simulink model "SigProcess"  (R2022b)
settings: Solver=FixedStepDiscrete  StartTime=0.0  StopTime=10.0  FixedStep=0.001  RelTol=1e-3
undefined symbols (not defined in the file): cClCddAdc_D_u16ADNum, cClCddAdc_D_u8FilterType, cClCddAdc_D_u8RawValueNum, cTmAfCtrl_Te_s32ShttrPosnColdOnHp
libraries: simulink x132
(part 7 of 7)

== system SigProcess/SigProcessSub/Stp5_ChangeAttrAndName/3_createPortGotoUpdate2/31_AdFilter/319_AVG5 ==
  sigin : Inport
  3191_MATLAB Function : MATLAB Function  TreatAsAtomicUnit=on
  Compare To Constant : simulink/Logic and Bit Operations/Compare To Constant  relop===  const=0  OutDataTypeStr=boolean
  Constant : Constant  Value=cClCddAdc_D_u8FilterType  OutDataTypeStr=uint8
  Constant1 : Constant  Value=cClCddAdc_D_u8RawValueNum  OutDataTypeStr=uint8
  Counter Limited : simulink/Sources/Counter Limited  uplimit=cClCddAdc_D_u8RawValueNum-1  tsamp=-1
  Data Store Memory : DataStoreMemory  DataStoreName=RecFlapFbRaw  ReadBeforeWriteMsg=warning  WriteAfterWriteMsg=warning  WriteAfterReadMsg=warning  ShowAdditionalParam=off  OutDataTypeStr=single  Dimensions=[1 20]
      settings: CopyFcn=set_param(gcbh,'ShowName','off');
  Data Store Read : DataStoreRead  DataStoreName=RecFlapFbRaw  IndexOptions=Index vector (dialog)  Indices=1  OutputSizes=1
  Data Store Write : DataStoreWrite  DataStoreName=RecFlapFbRaw  DataStoreElements=RecFlapFbRaw  EnableIndexing=on  IndexMode=Zero-based  IndexOptions=Index vector (port)  Indices=1  OutputSizes=1
  Data Type Conversion : DataTypeConversion  OutDataTypeStr=single  SaturateOnIntegerOverflow=off  RndMeth=Floor
  Gain1 : Gain  Gain=1/cClCddAdc_D_u8RawValueNum
  Multiport Switch : MultiPortSwitch  DataPortOrder=Zero-based contiguous  Inputs=5  DataPortForDefault=Additional data port  zeroidx=on  OutDataTypeStr=single  SaturateOnIntegerOverflow=off  InputSameDT=off
  Scope : Scope
  Sum of Elements1 : Sum  Inputs=+
  Switch : Switch  Criteria=u2 ~= 0  SaturateOnIntegerOverflow=off  InputSameDT=off
  Unit Delay : UnitDelay  SampleTime=-1  HasFrameUpgradeWarning=on
  sigAvg : Outport  OutDataTypeStr=single
  wires:
  Constant1/1 -> 3191_MATLAB Function/2(num)
  [sigAvg] -> sigAvg/1
  Multiport Switch/1 -> [sigAvg]
  [siginSingle] -> Multiport Switch/2
  [sigAvgQuick] -> Multiport Switch/6
  [sigAvgSimple] -> Multiport Switch/5
  [sigAvgSortWithoutEdge] -> Multiport Switch/4
  [sigAvgSortedMid] -> Multiport Switch/3
  Constant/1 -> Multiport Switch/1
  [sigin] -> Multiport Switch/7
  [sigin] -> Data Type Conversion/1
  sigin/1 -> [sigin]
  3191_MATLAB Function/1(mid) -> [sigAvgSortedMid]
  Unit Delay/1 -> Switch/3
  3191_MATLAB Function/2(withoutEdge) -> [sigAvgSortWithoutEdge]
  Data Type Conversion/1 -> Scope/1, Data Store Write/1, [siginSingle]
  Counter Limited/1 -> Data Store Write/2, Compare To Constant/1
  Gain1/1 -> [sigAvgQuick], Switch/1
  Switch/1 -> Unit Delay/1, [sigAvgSimple]
  Compare To Constant/1 -> Switch/2
  Sum of Elements1/1 -> Gain1/1
  Data Store Read/1 -> Sum of Elements1/1, 3191_MATLAB Function/1(u)

== system SigProcess/SigProcessSub/Stp5_ChangeAttrAndName/1_createPortGotoUpdate/11_AdFilter/113_AVG/1131_Ad2Volt ==
  ad : Inport
  Gain : Gain  Gain=5/cClCddAdc_D_u16ADNum
  volt : Outport
  wires:
  ad/1 -> Gain/1
  Gain/1 -> volt/1

== system SigProcess/SigProcessSub/Stp5_ChangeAttrAndName/2_createPortGotoUpdate1/21_AdFilter/213_AVG/2131_Ad2Volt ==
  ad : Inport
  Gain : Gain  Gain=5/cClCddAdc_D_u16ADNum
  volt : Outport
  wires:
  Gain/1 -> volt/1
  ad/1 -> Gain/1

== system SigProcess/SigProcessSub/Stp5_ChangeAttrAndName/3_createPortGotoUpdate2/31_AdFilter/313_AVG/3131_Ad2Volt ==
  ad : Inport
  Gain : Gain  Gain=5/cClCddAdc_D_u16ADNum
  volt : Outport
  wires:
  ad/1 -> Gain/1
  Gain/1 -> volt/1

== matlab function SigProcess/SigProcessSub/Stp3_createGotoUpdate/CLHB02001_AdFilter/AVG1/MATLAB Function ==
  data: u input; mid output; withoutEdge output; num input

function [mid, withoutEdge] = fcn(u,num)
% 输入u: 待排序数组
% 输入num: 滤波个数，max is 20
n = num;
for i = 1:n-1
    for j = 1:n-i
        if u(j) > u(j+1)
            temp = u(j);
            u(j) = u(j+1);
            u(j+1) = temp;
        end
    end
end
sortedData = u;

mid = sortedData(ceil(num/2)); % 取中间值
withoutEdge = mean(sortedData(2:num-1));

== matlab function SigProcess/SigProcessSub/Stp3_createGotoUpdate/CLHB02001_AdFilter/AVG10/MATLAB Function ==
  data: u input; mid output; withoutEdge output; num input

function [mid, withoutEdge] = fcn(u,num)
% 输入u: 待排序数组
% 输入num: 滤波个数，max is 20
n = num;
for i = 1:n-1
    for j = 1:n-i
        if u(j) > u(j+1)
            temp = u(j);
            u(j) = u(j+1);
            u(j+1) = temp;
        end
    end
end
sortedData = u;

mid = sortedData(ceil(num/2)); % 取中间值
withoutEdge = mean(sortedData(2:num-1));

== matlab function SigProcess/SigProcessSub/Stp4_createSubModInfo/CLHB02001_AdFilter/AVG/MATLAB Function ==
  data: u input; mid output; withoutEdge output; num input

function [mid, withoutEdge] = fcn(u,num)
% 输入u: 待排序数组
% 输入num: 滤波个数，max is 20
n = num;
for i = 1:n-1
    for j = 1:n-i
        if u(j) > u(j+1)
            temp = u(j);
            u(j) = u(j+1);
            u(j+1) = temp;
        end
    end
end
sortedData = u;

mid = sortedData(ceil(num/2)); % 取中间值
withoutEdge = mean(sortedData(2:num-1));

== matlab function SigProcess/SigProcessSub/Stp4_createSubModInfo/CLHB02001_AdFilter/AVG1/MATLAB Function ==
  data: u input; mid output; withoutEdge output; num input

function [mid, withoutEdge] = fcn(u,num)
% 输入u: 待排序数组
% 输入num: 滤波个数，max is 20
n = num;
for i = 1:n-1
    for j = 1:n-i
        if u(j) > u(j+1)
            temp = u(j);
            u(j) = u(j+1);
            u(j+1) = temp;
        end
    end
end
sortedData = u;

mid = sortedData(ceil(num/2)); % 取中间值
withoutEdge = mean(sortedData(2:num-1));

== matlab function SigProcess/SigProcessSub/Stp4_createSubModInfo/CLHB02001_AdFilter/AVG10/MATLAB Function ==
  data: u input; mid output; withoutEdge output; num input

function [mid, withoutEdge] = fcn(u,num)
% 输入u: 待排序数组
% 输入num: 滤波个数，max is 20
n = num;
for i = 1:n-1
    for j = 1:n-i
        if u(j) > u(j+1)
            temp = u(j);
            u(j) = u(j+1);
            u(j+1) = temp;
        end
    end
end
sortedData = u;

mid = sortedData(ceil(num/2)); % 取中间值
withoutEdge = mean(sortedData(2:num-1));

== matlab function SigProcess/SigProcessSub/Stp4_createSubModInfo/CLHB02001_AdFilter/AVG2/MATLAB Function ==
  data: u input; mid output; withoutEdge output; num input

function [mid, withoutEdge] = fcn(u,num)
% 输入u: 待排序数组
% 输入num: 滤波个数，max is 20
n = num;
for i = 1:n-1
    for j = 1:n-i
        if u(j) > u(j+1)
            temp = u(j);
            u(j) = u(j+1);
            u(j+1) = temp;
        end
    end
end
sortedData = u;

mid = sortedData(ceil(num/2)); % 取中间值
withoutEdge = mean(sortedData(2:num-1));

== matlab function SigProcess/SigProcessSub/Stp4_createSubModInfo/CLHB02001_AdFilter/AVG3/MATLAB Function ==
  data: u input; mid output; withoutEdge output; num input

function [mid, withoutEdge] = fcn(u,num)
% 输入u: 待排序数组
% 输入num: 滤波个数，max is 20
n = num;
for i = 1:n-1
    for j = 1:n-i
        if u(j) > u(j+1)
            temp = u(j);
            u(j) = u(j+1);
            u(j+1) = temp;
        end
    end
end
sortedData = u;

mid = sortedData(ceil(num/2)); % 取中间值
withoutEdge = mean(sortedData(2:num-1));

== matlab function SigProcess/SigProcessSub/Stp4_createSubModInfo/CLHB02001_AdFilter/AVG4/MATLAB Function ==
  data: u input; mid output; withoutEdge output; num input

function [mid, withoutEdge] = fcn(u,num)
% 输入u: 待排序数组
% 输入num: 滤波个数，max is 20
n = num;
for i = 1:n-1
    for j = 1:n-i
        if u(j) > u(j+1)
            temp = u(j);
            u(j) = u(j+1);
            u(j+1) = temp;
        end
    end
end
sortedData = u;

mid = sortedData(ceil(num/2)); % 取中间值
withoutEdge = mean(sortedData(2:num-1));

== matlab function SigProcess/SigProcessSub/Stp4_createSubModInfo/CLHB02001_AdFilter/AVG5/MATLAB Function ==
  data: u input; mid output; withoutEdge output; num input

function [mid, withoutEdge] = fcn(u,num)
% 输入u: 待排序数组
% 输入num: 滤波个数，max is 20
n = num;
for i = 1:n-1
    for j = 1:n-i
        if u(j) > u(j+1)
            temp = u(j);
            u(j) = u(j+1);
            u(j+1) = temp;
        end
    end
end
sortedData = u;

mid = sortedData(ceil(num/2)); % 取中间值
withoutEdge = mean(sortedData(2:num-1));

== matlab function SigProcess/SigProcessSub/Stp4_createSubModInfo/CLHB02001_AdFilter/AVG6/MATLAB Function ==
  data: u input; mid output; withoutEdge output; num input

function [mid, withoutEdge] = fcn(u,num)
% 输入u: 待排序数组
% 输入num: 滤波个数，max is 20
n = num;
for i = 1:n-1
    for j = 1:n-i
        if u(j) > u(j+1)
            temp = u(j);
            u(j) = u(j+1);
            u(j+1) = temp;
        end
    end
end
sortedData = u;

mid = sortedData(ceil(num/2)); % 取中间值
withoutEdge = mean(sortedData(2:num-1));

== matlab function SigProcess/SigProcessSub/Stp4_createSubModInfo/CLHB02001_AdFilter/AVG7/MATLAB Function ==
  data: u input; mid output; withoutEdge output; num input

function [mid, withoutEdge] = fcn(u,num)
% 输入u: 待排序数组
% 输入num: 滤波个数，max is 20
n = num;
for i = 1:n-1
    for j = 1:n-i
        if u(j) > u(j+1)
            temp = u(j);
            u(j) = u(j+1);
            u(j+1) = temp;
        end
    end
end
sortedData = u;

mid = sortedData(ceil(num/2)); % 取中间值
withoutEdge = mean(sortedData(2:num-1));

== matlab function SigProcess/SigProcessSub/Stp3_createGotoUpdate/CLHB02001_AdFilter/AVG/MATLAB Function ==
  data: u input; mid output; withoutEdge output; num input

function [mid, withoutEdge] = fcn(u,num)
% 输入u: 待排序数组
% 输入num: 滤波个数，max is 20
n = num;
for i = 1:n-1
    for j = 1:n-i
        if u(j) > u(j+1)
            temp = u(j);
            u(j) = u(j+1);
            u(j+1) = temp;
        end
    end
end
sortedData = u;

mid = sortedData(ceil(num/2)); % 取中间值
withoutEdge = mean(sortedData(2:num-1));

== matlab function SigProcess/SigProcessSub/Stp4_createSubModInfo/CLHB02001_AdFilter/AVG8/MATLAB Function ==
  data: u input; mid output; withoutEdge output; num input

function [mid, withoutEdge] = fcn(u,num)
% 输入u: 待排序数组
% 输入num: 滤波个数，max is 20
n = num;
for i = 1:n-1
    for j = 1:n-i
        if u(j) > u(j+1)
            temp = u(j);
            u(j) = u(j+1);
            u(j+1) = temp;
        end
    end
end
sortedData = u;

mid = sortedData(ceil(num/2)); % 取中间值
withoutEdge = mean(sortedData(2:num-1));

== matlab function SigProcess/SigProcessSub/Stp4_createSubModInfo/CLHB02001_AdFilter/AVG9/MATLAB Function ==
  data: u input; mid output; withoutEdge output; num input

function [mid, withoutEdge] = fcn(u,num)
% 输入u: 待排序数组
% 输入num: 滤波个数，max is 20
n = num;
for i = 1:n-1
    for j = 1:n-i
        if u(j) > u(j+1)
            temp = u(j);
            u(j) = u(j+1);
            u(j+1) = temp;
        end
    end
end
sortedData = u;

mid = sortedData(ceil(num/2)); % 取中间值
withoutEdge = mean(sortedData(2:num-1));

== matlab function SigProcess/SigProcessSub/Stp6_createPortGotoUpdate/CLHB02001_AdFilter/AVG/MATLAB Function ==
  data: u input; mid output; withoutEdge output; num input

function [mid, withoutEdge] = fcn(u,num)
% 输入u: 待排序数组
% 输入num: 滤波个数，max is 20
n = num;
for i = 1:n-1
    for j = 1:n-i
        if u(j) > u(j+1)
            temp = u(j);
            u(j) = u(j+1);
            u(j+1) = temp;
        end
    end
end
sortedData = u;

mid = sortedData(ceil(num/2)); % 取中间值
withoutEdge = mean(sortedData(2:num-1));

== matlab function SigProcess/SigProcessSub/Stp6_createPortGotoUpdate/CLHB02001_AdFilter/AVG1/MATLAB Function ==
  data: u input; mid output; withoutEdge output; num input

function [mid, withoutEdge] = fcn(u,num)
% 输入u: 待排序数组
% 输入num: 滤波个数，max is 20
n = num;
for i = 1:n-1
    for j = 1:n-i
        if u(j) > u(j+1)
            temp = u(j);
            u(j) = u(j+1);
            u(j+1) = temp;
        end
    end
end
sortedData = u;

mid = sortedData(ceil(num/2)); % 取中间值
withoutEdge = mean(sortedData(2:num-1));

== matlab function SigProcess/SigProcessSub/Stp6_createPortGotoUpdate/CLHB02001_AdFilter/AVG10/MATLAB Function ==
  data: u input; mid output; withoutEdge output; num input

function [mid, withoutEdge] = fcn(u,num)
% 输入u: 待排序数组
% 输入num: 滤波个数，max is 20
n = num;
for i = 1:n-1
    for j = 1:n-i
        if u(j) > u(j+1)
            temp = u(j);
            u(j) = u(j+1);
            u(j+1) = temp;
        end
    end
end
sortedData = u;

mid = sortedData(ceil(num/2)); % 取中间值
withoutEdge = mean(sortedData(2:num-1));

== matlab function SigProcess/SigProcessSub/Stp6_createPortGotoUpdate/CLHB02001_AdFilter/AVG2/MATLAB Function ==
  data: u input; mid output; withoutEdge output; num input

function [mid, withoutEdge] = fcn(u,num)
% 输入u: 待排序数组
% 输入num: 滤波个数，max is 20
n = num;
for i = 1:n-1
    for j = 1:n-i
        if u(j) > u(j+1)
            temp = u(j);
            u(j) = u(j+1);
            u(j+1) = temp;
        end
    end
end
sortedData = u;

mid = sortedData(ceil(num/2)); % 取中间值
withoutEdge = mean(sortedData(2:num-1));

== matlab function SigProcess/SigProcessSub/Stp6_createPortGotoUpdate/CLHB02001_AdFilter/AVG3/MATLAB Function ==
  data: u input; mid output; withoutEdge output; num input

function [mid, withoutEdge] = fcn(u,num)
% 输入u: 待排序数组
% 输入num: 滤波个数，max is 20
n = num;
for i = 1:n-1
    for j = 1:n-i
        if u(j) > u(j+1)
            temp = u(j);
            u(j) = u(j+1);
            u(j+1) = temp;
        end
    end
end
sortedData = u;

mid = sortedData(ceil(num/2)); % 取中间值
withoutEdge = mean(sortedData(2:num-1));

== matlab function SigProcess/SigProcessSub/Stp6_createPortGotoUpdate/CLHB02001_AdFilter/AVG4/MATLAB Function ==
  data: u input; mid output; withoutEdge output; num input

function [mid, withoutEdge] = fcn(u,num)
% 输入u: 待排序数组
% 输入num: 滤波个数，max is 20
n = num;
for i = 1:n-1
    for j = 1:n-i
        if u(j) > u(j+1)
            temp = u(j);
            u(j) = u(j+1);
            u(j+1) = temp;
        end
    end
end
sortedData = u;

mid = sortedData(ceil(num/2)); % 取中间值
withoutEdge = mean(sortedData(2:num-1));

== matlab function SigProcess/SigProcessSub/Stp6_createPortGotoUpdate/CLHB02001_AdFilter/AVG5/MATLAB Function ==
  data: u input; mid output; withoutEdge output; num input

function [mid, withoutEdge] = fcn(u,num)
% 输入u: 待排序数组
% 输入num: 滤波个数，max is 20
n = num;
for i = 1:n-1
    for j = 1:n-i
        if u(j) > u(j+1)
            temp = u(j);
            u(j) = u(j+1);
            u(j+1) = temp;
        end
    end
end
sortedData = u;

mid = sortedData(ceil(num/2)); % 取中间值
withoutEdge = mean(sortedData(2:num-1));

== matlab function SigProcess/SigProcessSub/Stp6_createPortGotoUpdate/CLHB02001_AdFilter/AVG6/MATLAB Function ==
  data: u input; mid output; withoutEdge output; num input

function [mid, withoutEdge] = fcn(u,num)
% 输入u: 待排序数组
% 输入num: 滤波个数，max is 20
n = num;
for i = 1:n-1
    for j = 1:n-i
        if u(j) > u(j+1)
            temp = u(j);
            u(j) = u(j+1);
            u(j+1) = temp;
        end
    end
end
sortedData = u;

mid = sortedData(ceil(num/2)); % 取中间值
withoutEdge = mean(sortedData(2:num-1));

== matlab function SigProcess/SigProcessSub/Stp3_createGotoUpdate/CLHB02001_AdFilter/AVG2/MATLAB Function ==
  data: u input; mid output; withoutEdge output; num input

function [mid, withoutEdge] = fcn(u,num)
% 输入u: 待排序数组
% 输入num: 滤波个数，max is 20
n = num;
for i = 1:n-1
    for j = 1:n-i
        if u(j) > u(j+1)
            temp = u(j);
            u(j) = u(j+1);
            u(j+1) = temp;
        end
    end
end
sortedData = u;

mid = sortedData(ceil(num/2)); % 取中间值
withoutEdge = mean(sortedData(2:num-1));

== matlab function SigProcess/SigProcessSub/Stp6_createPortGotoUpdate/CLHB02001_AdFilter/AVG7/MATLAB Function ==
  data: u input; mid output; withoutEdge output; num input

function [mid, withoutEdge] = fcn(u,num)
% 输入u: 待排序数组
% 输入num: 滤波个数，max is 20
n = num;
for i = 1:n-1
    for j = 1:n-i
        if u(j) > u(j+1)
            temp = u(j);
            u(j) = u(j+1);
            u(j+1) = temp;
        end
    end
end
sortedData = u;

mid = sortedData(ceil(num/2)); % 取中间值
withoutEdge = mean(sortedData(2:num-1));

== matlab function SigProcess/SigProcessSub/Stp6_createPortGotoUpdate/CLHB02001_AdFilter/AVG8/MATLAB Function ==
  data: u input; mid output; withoutEdge output; num input

function [mid, withoutEdge] = fcn(u,num)
% 输入u: 待排序数组
% 输入num: 滤波个数，max is 20
n = num;
for i = 1:n-1
    for j = 1:n-i
        if u(j) > u(j+1)
            temp = u(j);
            u(j) = u(j+1);
            u(j+1) = temp;
        end
    end
end
sortedData = u;

mid = sortedData(ceil(num/2)); % 取中间值
withoutEdge = mean(sortedData(2:num-1));

== matlab function SigProcess/SigProcessSub/Stp6_createPortGotoUpdate/CLHB02001_AdFilter/AVG9/MATLAB Function ==
  data: u input; mid output; withoutEdge output; num input

function [mid, withoutEdge] = fcn(u,num)
% 输入u: 待排序数组
% 输入num: 滤波个数，max is 20
n = num;
for i = 1:n-1
    for j = 1:n-i
        if u(j) > u(j+1)
            temp = u(j);
            u(j) = u(j+1);
            u(j+1) = temp;
        end
    end
end
sortedData = u;

mid = sortedData(ceil(num/2)); % 取中间值
withoutEdge = mean(sortedData(2:num-1));

== matlab function SigProcess/SigProcessSub/Stp5_ChangeAttrAndName/2_createPortGotoUpdate1/21_AdFilter/213_AVG/2132_MATLAB Function ==
  data: u input; mid output; withoutEdge output; num input

function [mid, withoutEdge] = fcn(u,num)
% 输入u: 待排序数组
% 输入num: 滤波个数，max is 20
n = num;
for i = 1:n-1
    for j = 1:n-i
        if u(j) > u(j+1)
            temp = u(j);
            u(j) = u(j+1);
            u(j+1) = temp;
        end
    end
end
sortedData = u;

mid = sortedData(ceil(num/2)); % 取中间值
withoutEdge = mean(sortedData(2:num-1));

== matlab function SigProcess/SigProcessSub/Stp5_ChangeAttrAndName/2_createPortGotoUpdate1/21_AdFilter/214_AVG1/2141_MATLAB Function ==
  data: u input; mid output; withoutEdge output; num input

function [mid, withoutEdge] = fcn(u,num)
% 输入u: 待排序数组
% 输入num: 滤波个数，max is 20
n = num;
for i = 1:n-1
    for j = 1:n-i
        if u(j) > u(j+1)
            temp = u(j);
            u(j) = u(j+1);
            u(j+1) = temp;
        end
    end
end
sortedData = u;

mid = sortedData(ceil(num/2)); % 取中间值
withoutEdge = mean(sortedData(2:num-1));

== matlab function SigProcess/SigProcessSub/Stp5_ChangeAttrAndName/2_createPortGotoUpdate1/21_AdFilter/215_AVG10/2151_MATLAB Function ==
  data: u input; mid output; withoutEdge output; num input

function [mid, withoutEdge] = fcn(u,num)
% 输入u: 待排序数组
% 输入num: 滤波个数，max is 20
n = num;
for i = 1:n-1
    for j = 1:n-i
        if u(j) > u(j+1)
            temp = u(j);
            u(j) = u(j+1);
            u(j+1) = temp;
        end
    end
end
sortedData = u;

mid = sortedData(ceil(num/2)); % 取中间值
withoutEdge = mean(sortedData(2:num-1));

== matlab function SigProcess/SigProcessSub/Stp5_ChangeAttrAndName/2_createPortGotoUpdate1/21_AdFilter/216_AVG2/2161_MATLAB Function ==
  data: u input; mid output; withoutEdge output; num input

function [mid, withoutEdge] = fcn(u,num)
% 输入u: 待排序数组
% 输入num: 滤波个数，max is 20
n = num;
for i = 1:n-1
    for j = 1:n-i
        if u(j) > u(j+1)
            temp = u(j);
            u(j) = u(j+1);
            u(j+1) = temp;
        end
    end
end
sortedData = u;

mid = sortedData(ceil(num/2)); % 取中间值
withoutEdge = mean(sortedData(2:num-1));

== matlab function SigProcess/SigProcessSub/Stp5_ChangeAttrAndName/2_createPortGotoUpdate1/21_AdFilter/217_AVG3/2171_MATLAB Function ==
  data: u input; mid output; withoutEdge output; num input

function [mid, withoutEdge] = fcn(u,num)
% 输入u: 待排序数组
% 输入num: 滤波个数，max is 20
n = num;
for i = 1:n-1
    for j = 1:n-i
        if u(j) > u(j+1)
            temp = u(j);
            u(j) = u(j+1);
            u(j+1) = temp;
        end
    end
end
sortedData = u;

mid = sortedData(ceil(num/2)); % 取中间值
withoutEdge = mean(sortedData(2:num-1));

== matlab function SigProcess/SigProcessSub/Stp5_ChangeAttrAndName/2_createPortGotoUpdate1/21_AdFilter/218_AVG4/2181_MATLAB Function ==
  data: u input; mid output; withoutEdge output; num input

function [mid, withoutEdge] = fcn(u,num)
% 输入u: 待排序数组
% 输入num: 滤波个数，max is 20
n = num;
for i = 1:n-1
    for j = 1:n-i
        if u(j) > u(j+1)
            temp = u(j);
            u(j) = u(j+1);
            u(j+1) = temp;
        end
    end
end
sortedData = u;

mid = sortedData(ceil(num/2)); % 取中间值
withoutEdge = mean(sortedData(2:num-1));

== matlab function SigProcess/SigProcessSub/Stp5_ChangeAttrAndName/2_createPortGotoUpdate1/21_AdFilter/219_AVG5/2191_MATLAB Function ==
  data: u input; mid output; withoutEdge output; num input

function [mid, withoutEdge] = fcn(u,num)
% 输入u: 待排序数组
% 输入num: 滤波个数，max is 20
n = num;
for i = 1:n-1
    for j = 1:n-i
        if u(j) > u(j+1)
            temp = u(j);
            u(j) = u(j+1);
            u(j+1) = temp;
        end
    end
end
sortedData = u;

mid = sortedData(ceil(num/2)); % 取中间值
withoutEdge = mean(sortedData(2:num-1));

== matlab function SigProcess/SigProcessSub/Stp3_createGotoUpdate/CLHB02001_AdFilter/AVG3/MATLAB Function ==
  data: u input; mid output; withoutEdge output; num input

function [mid, withoutEdge] = fcn(u,num)
% 输入u: 待排序数组
% 输入num: 滤波个数，max is 20
n = num;
for i = 1:n-1
    for j = 1:n-i
        if u(j) > u(j+1)
            temp = u(j);
            u(j) = u(j+1);
            u(j+1) = temp;
        end
    end
end
sortedData = u;

mid = sortedData(ceil(num/2)); % 取中间值
withoutEdge = mean(sortedData(2:num-1));

== matlab function SigProcess/SigProcessSub/Stp5_ChangeAttrAndName/2_createPortGotoUpdate1/21_AdFilter/2110_AVG6/21101_MATLAB Function ==
  data: u input; mid output; withoutEdge output; num input

function [mid, withoutEdge] = fcn(u,num)
% 输入u: 待排序数组
% 输入num: 滤波个数，max is 20
n = num;
for i = 1:n-1
    for j = 1:n-i
        if u(j) > u(j+1)
            temp = u(j);
            u(j) = u(j+1);
            u(j+1) = temp;
        end
    end
end
sortedData = u;

mid = sortedData(ceil(num/2)); % 取中间值
withoutEdge = mean(sortedData(2:num-1));

== matlab function SigProcess/SigProcessSub/Stp5_ChangeAttrAndName/2_createPortGotoUpdate1/21_AdFilter/2111_AVG7/21111_MATLAB Function ==
  data: u input; mid output; withoutEdge output; num input

function [mid, withoutEdge] = fcn(u,num)
% 输入u: 待排序数组
% 输入num: 滤波个数，max is 20
n = num;
for i = 1:n-1
    for j = 1:n-i
        if u(j) > u(j+1)
            temp = u(j);
            u(j) = u(j+1);
            u(j+1) = temp;
        end
    end
end
sortedData = u;

mid = sortedData(ceil(num/2)); % 取中间值
withoutEdge = mean(sortedData(2:num-1));

== matlab function SigProcess/SigProcessSub/Stp5_ChangeAttrAndName/2_createPortGotoUpdate1/21_AdFilter/211_AVG8/2111_MATLAB Function ==
  data: u input; mid output; withoutEdge output; num input

function [mid, withoutEdge] = fcn(u,num)
% 输入u: 待排序数组
% 输入num: 滤波个数，max is 20
n = num;
for i = 1:n-1
    for j = 1:n-i
        if u(j) > u(j+1)
            temp = u(j);
            u(j) = u(j+1);
            u(j+1) = temp;
        end
    end
end
sortedData = u;

mid = sortedData(ceil(num/2)); % 取中间值
withoutEdge = mean(sortedData(2:num-1));

== matlab function SigProcess/SigProcessSub/Stp5_ChangeAttrAndName/2_createPortGotoUpdate1/21_AdFilter/212_AVG9/2121_MATLAB Function ==
  data: u input; mid output; withoutEdge output; num input

function [mid, withoutEdge] = fcn(u,num)
% 输入u: 待排序数组
% 输入num: 滤波个数，max is 20
n = num;
for i = 1:n-1
    for j = 1:n-i
        if u(j) > u(j+1)
            temp = u(j);
            u(j) = u(j+1);
            u(j+1) = temp;
        end
    end
end
sortedData = u;

mid = sortedData(ceil(num/2)); % 取中间值
withoutEdge = mean(sortedData(2:num-1));

== matlab function SigProcess/SigProcessSub/Stp5_ChangeAttrAndName/1_createPortGotoUpdate/11_AdFilter/113_AVG/1132_MATLAB Function ==
  data: u input; mid output; withoutEdge output; num input

function [mid, withoutEdge] = fcn(u,num)
% 输入u: 待排序数组
% 输入num: 滤波个数，max is 20
n = num;
for i = 1:n-1
    for j = 1:n-i
        if u(j) > u(j+1)
            temp = u(j);
            u(j) = u(j+1);
            u(j+1) = temp;
        end
    end
end
sortedData = u;

mid = sortedData(ceil(num/2)); % 取中间值
withoutEdge = mean(sortedData(2:num-1));

== matlab function SigProcess/SigProcessSub/Stp5_ChangeAttrAndName/1_createPortGotoUpdate/11_AdFilter/114_AVG1/1141_MATLAB Function ==
  data: u input; mid output; withoutEdge output; num input

function [mid, withoutEdge] = fcn(u,num)
% 输入u: 待排序数组
% 输入num: 滤波个数，max is 20
n = num;
for i = 1:n-1
    for j = 1:n-i
        if u(j) > u(j+1)
            temp = u(j);
            u(j) = u(j+1);
            u(j+1) = temp;
        end
    end
end
sortedData = u;

mid = sortedData(ceil(num/2)); % 取中间值
withoutEdge = mean(sortedData(2:num-1));

== matlab function SigProcess/SigProcessSub/Stp5_ChangeAttrAndName/1_createPortGotoUpdate/11_AdFilter/115_AVG10/1151_MATLAB Function ==
  data: u input; mid output; withoutEdge output; num input

function [mid, withoutEdge] = fcn(u,num)
% 输入u: 待排序数组
% 输入num: 滤波个数，max is 20
n = num;
for i = 1:n-1
    for j = 1:n-i
        if u(j) > u(j+1)
            temp = u(j);
            u(j) = u(j+1);
            u(j+1) = temp;
        end
    end
end
sortedData = u;

mid = sortedData(ceil(num/2)); % 取中间值
withoutEdge = mean(sortedData(2:num-1));

== matlab function SigProcess/SigProcessSub/Stp5_ChangeAttrAndName/1_createPortGotoUpdate/11_AdFilter/116_AVG2/1161_MATLAB Function ==
  data: u input; mid output; withoutEdge output; num input

function [mid, withoutEdge] = fcn(u,num)
% 输入u: 待排序数组
% 输入num: 滤波个数，max is 20
n = num;
for i = 1:n-1
    for j = 1:n-i
        if u(j) > u(j+1)
            temp = u(j);
            u(j) = u(j+1);
            u(j+1) = temp;
        end
    end
end
sortedData = u;

mid = sortedData(ceil(num/2)); % 取中间值
withoutEdge = mean(sortedData(2:num-1));

== matlab function SigProcess/SigProcessSub/Stp5_ChangeAttrAndName/1_createPortGotoUpdate/11_AdFilter/117_AVG3/1171_MATLAB Function ==
  data: u input; mid output; withoutEdge output; num input

function [mid, withoutEdge] = fcn(u,num)
% 输入u: 待排序数组
% 输入num: 滤波个数，max is 20
n = num;
for i = 1:n-1
    for j = 1:n-i
        if u(j) > u(j+1)
            temp = u(j);
            u(j) = u(j+1);
            u(j+1) = temp;
        end
    end
end
sortedData = u;

mid = sortedData(ceil(num/2)); % 取中间值
withoutEdge = mean(sortedData(2:num-1));

== matlab function SigProcess/SigProcessSub/Stp5_ChangeAttrAndName/1_createPortGotoUpdate/11_AdFilter/118_AVG4/1181_MATLAB Function ==
  data: u input; mid output; withoutEdge output; num input

function [mid, withoutEdge] = fcn(u,num)
% 输入u: 待排序数组
% 输入num: 滤波个数，max is 20
n = num;
for i = 1:n-1
    for j = 1:n-i
        if u(j) > u(j+1)
            temp = u(j);
            u(j) = u(j+1);
            u(j+1) = temp;
        end
    end
end
sortedData = u;

mid = sortedData(ceil(num/2)); % 取中间值
withoutEdge = mean(sortedData(2:num-1));

== matlab function SigProcess/SigProcessSub/Stp3_createGotoUpdate/CLHB02001_AdFilter/AVG4/MATLAB Function ==
  data: u input; mid output; withoutEdge output; num input

function [mid, withoutEdge] = fcn(u,num)
% 输入u: 待排序数组
% 输入num: 滤波个数，max is 20
n = num;
for i = 1:n-1
    for j = 1:n-i
        if u(j) > u(j+1)
            temp = u(j);
            u(j) = u(j+1);
            u(j+1) = temp;
        end
    end
end
sortedData = u;

mid = sortedData(ceil(num/2)); % 取中间值
withoutEdge = mean(sortedData(2:num-1));

== matlab function SigProcess/SigProcessSub/Stp5_ChangeAttrAndName/1_createPortGotoUpdate/11_AdFilter/119_AVG5/1191_MATLAB Function ==
  data: u input; mid output; withoutEdge output; num input

function [mid, withoutEdge] = fcn(u,num)
% 输入u: 待排序数组
% 输入num: 滤波个数，max is 20
n = num;
for i = 1:n-1
    for j = 1:n-i
        if u(j) > u(j+1)
            temp = u(j);
            u(j) = u(j+1);
            u(j+1) = temp;
        end
    end
end
sortedData = u;

mid = sortedData(ceil(num/2)); % 取中间值
withoutEdge = mean(sortedData(2:num-1));

== matlab function SigProcess/SigProcessSub/Stp5_ChangeAttrAndName/1_createPortGotoUpdate/11_AdFilter/1110_AVG6/11101_MATLAB Function ==
  data: u input; mid output; withoutEdge output; num input

function [mid, withoutEdge] = fcn(u,num)
% 输入u: 待排序数组
% 输入num: 滤波个数，max is 20
n = num;
for i = 1:n-1
    for j = 1:n-i
        if u(j) > u(j+1)
            temp = u(j);
            u(j) = u(j+1);
            u(j+1) = temp;
        end
    end
end
sortedData = u;

mid = sortedData(ceil(num/2)); % 取中间值
withoutEdge = mean(sortedData(2:num-1));

== matlab function SigProcess/SigProcessSub/Stp5_ChangeAttrAndName/1_createPortGotoUpdate/11_AdFilter/1111_AVG7/11111_MATLAB Function ==
  data: u input; mid output; withoutEdge output; num input

function [mid, withoutEdge] = fcn(u,num)
% 输入u: 待排序数组
% 输入num: 滤波个数，max is 20
n = num;
for i = 1:n-1
    for j = 1:n-i
        if u(j) > u(j+1)
            temp = u(j);
            u(j) = u(j+1);
            u(j+1) = temp;
        end
    end
end
sortedData = u;

mid = sortedData(ceil(num/2)); % 取中间值
withoutEdge = mean(sortedData(2:num-1));

== matlab function SigProcess/SigProcessSub/Stp5_ChangeAttrAndName/1_createPortGotoUpdate/11_AdFilter/111_AVG8/1111_MATLAB Function ==
  data: u input; mid output; withoutEdge output; num input

function [mid, withoutEdge] = fcn(u,num)
% 输入u: 待排序数组
% 输入num: 滤波个数，max is 20
n = num;
for i = 1:n-1
    for j = 1:n-i
        if u(j) > u(j+1)
            temp = u(j);
            u(j) = u(j+1);
            u(j+1) = temp;
        end
    end
end
sortedData = u;

mid = sortedData(ceil(num/2)); % 取中间值
withoutEdge = mean(sortedData(2:num-1));

== matlab function SigProcess/SigProcessSub/Stp5_ChangeAttrAndName/1_createPortGotoUpdate/11_AdFilter/112_AVG9/1121_MATLAB Function ==
  data: u input; mid output; withoutEdge output; num input

function [mid, withoutEdge] = fcn(u,num)
% 输入u: 待排序数组
% 输入num: 滤波个数，max is 20
n = num;
for i = 1:n-1
    for j = 1:n-i
        if u(j) > u(j+1)
            temp = u(j);
            u(j) = u(j+1);
            u(j+1) = temp;
        end
    end
end
sortedData = u;

mid = sortedData(ceil(num/2)); % 取中间值
withoutEdge = mean(sortedData(2:num-1));

== matlab function SigProcess/SigProcessSub/Stp5_ChangeAttrAndName/3_createPortGotoUpdate2/31_AdFilter/313_AVG/3132_MATLAB Function ==
  data: u input; mid output; withoutEdge output; num input

function [mid, withoutEdge] = fcn(u,num)
% 输入u: 待排序数组
% 输入num: 滤波个数，max is 20
n = num;
for i = 1:n-1
    for j = 1:n-i
        if u(j) > u(j+1)
            temp = u(j);
            u(j) = u(j+1);
            u(j+1) = temp;
        end
    end
end
sortedData = u;

mid = sortedData(ceil(num/2)); % 取中间值
withoutEdge = mean(sortedData(2:num-1));

== matlab function SigProcess/SigProcessSub/Stp5_ChangeAttrAndName/3_createPortGotoUpdate2/31_AdFilter/314_AVG1/3141_MATLAB Function ==
  data: u input; mid output; withoutEdge output; num input

function [mid, withoutEdge] = fcn(u,num)
% 输入u: 待排序数组
% 输入num: 滤波个数，max is 20
n = num;
for i = 1:n-1
    for j = 1:n-i
        if u(j) > u(j+1)
            temp = u(j);
            u(j) = u(j+1);
            u(j+1) = temp;
        end
    end
end
sortedData = u;

mid = sortedData(ceil(num/2)); % 取中间值
withoutEdge = mean(sortedData(2:num-1));

== matlab function SigProcess/SigProcessSub/Stp5_ChangeAttrAndName/3_createPortGotoUpdate2/31_AdFilter/315_AVG10/3151_MATLAB Function ==
  data: u input; mid output; withoutEdge output; num input

function [mid, withoutEdge] = fcn(u,num)
% 输入u: 待排序数组
% 输入num: 滤波个数，max is 20
n = num;
for i = 1:n-1
    for j = 1:n-i
        if u(j) > u(j+1)
            temp = u(j);
            u(j) = u(j+1);
            u(j+1) = temp;
        end
    end
end
sortedData = u;

mid = sortedData(ceil(num/2)); % 取中间值
withoutEdge = mean(sortedData(2:num-1));

== matlab function SigProcess/SigProcessSub/Stp5_ChangeAttrAndName/3_createPortGotoUpdate2/31_AdFilter/316_AVG2/3161_MATLAB Function ==
  data: u input; mid output; withoutEdge output; num input

function [mid, withoutEdge] = fcn(u,num)
% 输入u: 待排序数组
% 输入num: 滤波个数，max is 20
n = num;
for i = 1:n-1
    for j = 1:n-i
        if u(j) > u(j+1)
            temp = u(j);
            u(j) = u(j+1);
            u(j+1) = temp;
        end
    end
end
sortedData = u;

mid = sortedData(ceil(num/2)); % 取中间值
withoutEdge = mean(sortedData(2:num-1));

== matlab function SigProcess/SigProcessSub/Stp5_ChangeAttrAndName/3_createPortGotoUpdate2/31_AdFilter/317_AVG3/3171_MATLAB Function ==
  data: u input; mid output; withoutEdge output; num input

function [mid, withoutEdge] = fcn(u,num)
% 输入u: 待排序数组
% 输入num: 滤波个数，max is 20
n = num;
for i = 1:n-1
    for j = 1:n-i
        if u(j) > u(j+1)
            temp = u(j);
            u(j) = u(j+1);
            u(j+1) = temp;
        end
    end
end
sortedData = u;

mid = sortedData(ceil(num/2)); % 取中间值
withoutEdge = mean(sortedData(2:num-1));

== matlab function SigProcess/SigProcessSub/Stp3_createGotoUpdate/CLHB02001_AdFilter/AVG5/MATLAB Function ==
  data: u input; mid output; withoutEdge output; num input

function [mid, withoutEdge] = fcn(u,num)
% 输入u: 待排序数组
% 输入num: 滤波个数，max is 20
n = num;
for i = 1:n-1
    for j = 1:n-i
        if u(j) > u(j+1)
            temp = u(j);
            u(j) = u(j+1);
            u(j+1) = temp;
        end
    end
end
sortedData = u;

mid = sortedData(ceil(num/2)); % 取中间值
withoutEdge = mean(sortedData(2:num-1));

== matlab function SigProcess/SigProcessSub/Stp5_ChangeAttrAndName/3_createPortGotoUpdate2/31_AdFilter/318_AVG4/3181_MATLAB Function ==
  data: u input; mid output; withoutEdge output; num input

function [mid, withoutEdge] = fcn(u,num)
% 输入u: 待排序数组
% 输入num: 滤波个数，max is 20
n = num;
for i = 1:n-1
    for j = 1:n-i
        if u(j) > u(j+1)
            temp = u(j);
            u(j) = u(j+1);
            u(j+1) = temp;
        end
    end
end
sortedData = u;

mid = sortedData(ceil(num/2)); % 取中间值
withoutEdge = mean(sortedData(2:num-1));

== matlab function SigProcess/SigProcessSub/Stp5_ChangeAttrAndName/3_createPortGotoUpdate2/31_AdFilter/319_AVG5/3191_MATLAB Function ==
  data: u input; mid output; withoutEdge output; num input

function [mid, withoutEdge] = fcn(u,num)
% 输入u: 待排序数组
% 输入num: 滤波个数，max is 20
n = num;
for i = 1:n-1
    for j = 1:n-i
        if u(j) > u(j+1)
            temp = u(j);
            u(j) = u(j+1);
            u(j+1) = temp;
        end
    end
end
sortedData = u;

mid = sortedData(ceil(num/2)); % 取中间值
withoutEdge = mean(sortedData(2:num-1));

== matlab function SigProcess/SigProcessSub/Stp5_ChangeAttrAndName/3_createPortGotoUpdate2/31_AdFilter/3110_AVG6/31101_MATLAB Function ==
  data: u input; mid output; withoutEdge output; num input

function [mid, withoutEdge] = fcn(u,num)
% 输入u: 待排序数组
% 输入num: 滤波个数，max is 20
n = num;
for i = 1:n-1
    for j = 1:n-i
        if u(j) > u(j+1)
            temp = u(j);
            u(j) = u(j+1);
            u(j+1) = temp;
        end
    end
end
sortedData = u;

mid = sortedData(ceil(num/2)); % 取中间值
withoutEdge = mean(sortedData(2:num-1));

== matlab function SigProcess/SigProcessSub/Stp5_ChangeAttrAndName/3_createPortGotoUpdate2/31_AdFilter/3111_AVG7/31111_MATLAB Function ==
  data: u input; mid output; withoutEdge output; num input

function [mid, withoutEdge] = fcn(u,num)
% 输入u: 待排序数组
% 输入num: 滤波个数，max is 20
n = num;
for i = 1:n-1
    for j = 1:n-i
        if u(j) > u(j+1)
            temp = u(j);
            u(j) = u(j+1);
            u(j+1) = temp;
        end
    end
end
sortedData = u;

mid = sortedData(ceil(num/2)); % 取中间值
withoutEdge = mean(sortedData(2:num-1));

== matlab function SigProcess/SigProcessSub/Stp5_ChangeAttrAndName/3_createPortGotoUpdate2/31_AdFilter/311_AVG8/3111_MATLAB Function ==
  data: u input; mid output; withoutEdge output; num input

function [mid, withoutEdge] = fcn(u,num)
% 输入u: 待排序数组
% 输入num: 滤波个数，max is 20
n = num;
for i = 1:n-1
    for j = 1:n-i
        if u(j) > u(j+1)
            temp = u(j);
            u(j) = u(j+1);
            u(j+1) = temp;
        end
    end
end
sortedData = u;

mid = sortedData(ceil(num/2)); % 取中间值
withoutEdge = mean(sortedData(2:num-1));

== matlab function SigProcess/SigProcessSub/Stp5_ChangeAttrAndName/3_createPortGotoUpdate2/31_AdFilter/312_AVG9/3121_MATLAB Function ==
  data: u input; mid output; withoutEdge output; num input

function [mid, withoutEdge] = fcn(u,num)
% 输入u: 待排序数组
% 输入num: 滤波个数，max is 20
n = num;
for i = 1:n-1
    for j = 1:n-i
        if u(j) > u(j+1)
            temp = u(j);
            u(j) = u(j+1);
            u(j+1) = temp;
        end
    end
end
sortedData = u;

mid = sortedData(ceil(num/2)); % 取中间值
withoutEdge = mean(sortedData(2:num-1));

== matlab function SigProcess/SigProcessSub/Stp3_createGotoUpdate/CLHB02001_AdFilter/AVG6/MATLAB Function ==
  data: u input; mid output; withoutEdge output; num input

function [mid, withoutEdge] = fcn(u,num)
% 输入u: 待排序数组
% 输入num: 滤波个数，max is 20
n = num;
for i = 1:n-1
    for j = 1:n-i
        if u(j) > u(j+1)
            temp = u(j);
            u(j) = u(j+1);
            u(j+1) = temp;
        end
    end
end
sortedData = u;

mid = sortedData(ceil(num/2)); % 取中间值
withoutEdge = mean(sortedData(2:num-1));

== matlab function SigProcess/SigProcessSub/Stp3_createGotoUpdate/CLHB02001_AdFilter/AVG7/MATLAB Function ==
  data: u input; mid output; withoutEdge output; num input

function [mid, withoutEdge] = fcn(u,num)
% 输入u: 待排序数组
% 输入num: 滤波个数，max is 20
n = num;
for i = 1:n-1
    for j = 1:n-i
        if u(j) > u(j+1)
            temp = u(j);
            u(j) = u(j+1);
            u(j+1) = temp;
        end
    end
end
sortedData = u;

mid = sortedData(ceil(num/2)); % 取中间值
withoutEdge = mean(sortedData(2:num-1));

== matlab function SigProcess/SigProcessSub/Stp3_createGotoUpdate/CLHB02001_AdFilter/AVG8/MATLAB Function ==
  data: u input; mid output; withoutEdge output; num input

function [mid, withoutEdge] = fcn(u,num)
% 输入u: 待排序数组
% 输入num: 滤波个数，max is 20
n = num;
for i = 1:n-1
    for j = 1:n-i
        if u(j) > u(j+1)
            temp = u(j);
            u(j) = u(j+1);
            u(j+1) = temp;
        end
    end
end
sortedData = u;

mid = sortedData(ceil(num/2)); % 取中间值
withoutEdge = mean(sortedData(2:num-1));

== matlab function SigProcess/SigProcessSub/Stp3_createGotoUpdate/CLHB02001_AdFilter/AVG9/MATLAB Function ==
  data: u input; mid output; withoutEdge output; num input

function [mid, withoutEdge] = fcn(u,num)
% 输入u: 待排序数组
% 输入num: 滤波个数，max is 20
n = num;
for i = 1:n-1
    for j = 1:n-i
        if u(j) > u(j+1)
            temp = u(j);
            u(j) = u(j+1);
            u(j+1) = temp;
        end
    end
end
sortedData = u;

mid = sortedData(ceil(num/2)); % 取中间值
withoutEdge = mean(sortedData(2:num-1));
